simulink model "robot_gripper_vr"  (Simulink 6.5)
settings: Solver=ode45  StartTime=0.0  StopTime=10  RelTol=1e-3
libraries: mblibv1 x39, vrlib x12
settings Model: Creator=arnav  LastModifiedBy=Danek

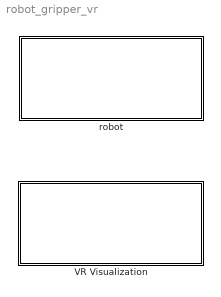
== system robot_gripper_vr ==
  VR Visualization : Subsystem
  robot : Subsystem

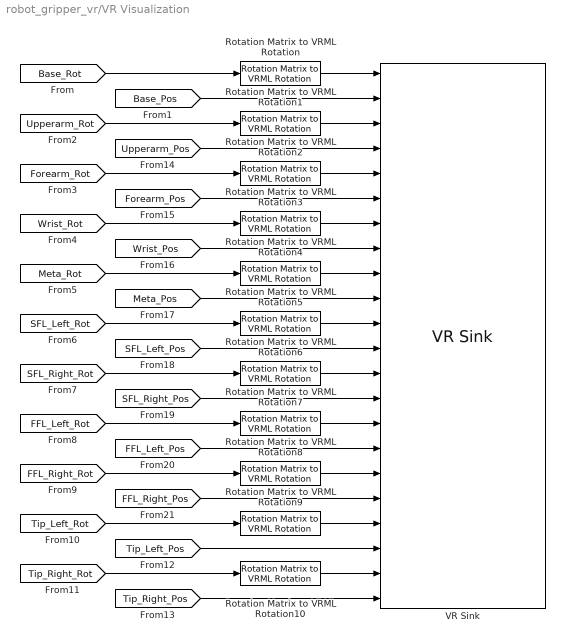
== system robot_gripper_vr/VR Visualization ==
  Rotation Matrix to VRML Rotation{,1..10} (11 alike) : vrlib/Utilities/Rotation Matrix to VRML Rotation  SystemSampleTime=-1  maxzero=1e-12
  VR Sink : vrlib/VR Sink  SampleTime=0.02  ViewEnable=on  RemoteChange=off  RemoteView=on  FieldsWritten=Base.rotation.4.1.double#Base.translation.3.1.double#Upperarm.rotation.4.1.double#Upperarm.translation.3.1.double#Forearm.rotation.4.1.double#Forearm.translation.3.1.double#Wrist.rotation.4.1.double#Wrist.translation.3.1.double#Metacarples.rotation.4.1.double#Metacarples.translation.3.1.double#Fingerlink2_Left.rotation.4.1.double#Fingerlink2_Left.translation.3.1.double#Fingerlink2_Right.rotation.4.1.double#Fingerlink2_Right.translation.3.1.double#Fingerlink1_Left.rotation.4.1.double#Fingerlink1_Left.translation.3.1.double#Fingerlink1_Right.rotation.4.1.double#Fingerlink1_Right.translation.3.1.double#Fingertip_Left.rotation.4.1.double#Fingertip_Left.translation.3.1.double#Fingertip_Right.rotation.4.1.double#Fingertip_Right.translation.3.1.double  WorldFileName=robot_gripper.wrl  WorldDescription=Robot Gripper  AutoView=off  FigureProperties={}
  wires:
  [Base_Rot] -> Rotation Matrix to VRML Rotation/1
  Rotation Matrix to VRML Rotation/1 -> VR Sink/1
  [Base_Pos] -> VR Sink/2
  [Upperarm_Rot] -> Rotation Matrix to VRML Rotation1/1
  [Forearm_Rot] -> Rotation Matrix to VRML Rotation2/1
  [Wrist_Rot] -> Rotation Matrix to VRML Rotation3/1
  [Meta_Rot] -> Rotation Matrix to VRML Rotation4/1
  [SFL_Left_Rot] -> Rotation Matrix to VRML Rotation5/1
  [SFL_Right_Rot] -> Rotation Matrix to VRML Rotation6/1
  [FFL_Left_Rot] -> Rotation Matrix to VRML Rotation7/1
  [FFL_Right_Rot] -> Rotation Matrix to VRML Rotation8/1
  [Tip_Left_Rot] -> Rotation Matrix to VRML Rotation9/1
  [Tip_Right_Rot] -> Rotation Matrix to VRML Rotation10/1
  Rotation Matrix to VRML Rotation1/1 -> VR Sink/3
  Rotation Matrix to VRML Rotation2/1 -> VR Sink/5
  Rotation Matrix to VRML Rotation3/1 -> VR Sink/7
  Rotation Matrix to VRML Rotation4/1 -> VR Sink/9
  Rotation Matrix to VRML Rotation5/1 -> VR Sink/11
  Rotation Matrix to VRML Rotation6/1 -> VR Sink/13
  Rotation Matrix to VRML Rotation7/1 -> VR Sink/15
  Rotation Matrix to VRML Rotation8/1 -> VR Sink/17
  Rotation Matrix to VRML Rotation9/1 -> VR Sink/19
  Rotation Matrix to VRML Rotation10/1 -> VR Sink/21
  [Upperarm_Pos] -> VR Sink/4
  [Forearm_Pos] -> VR Sink/6
  [Wrist_Pos] -> VR Sink/8
  [Meta_Pos] -> VR Sink/10
  [SFL_Left_Pos] -> VR Sink/12
  [SFL_Right_Pos] -> VR Sink/14
  [FFL_Left_Pos] -> VR Sink/16
  [FFL_Right_Pos] -> VR Sink/18
  [Tip_Left_Pos] -> VR Sink/20
  [Tip_Right_Pos] -> VR Sink/22

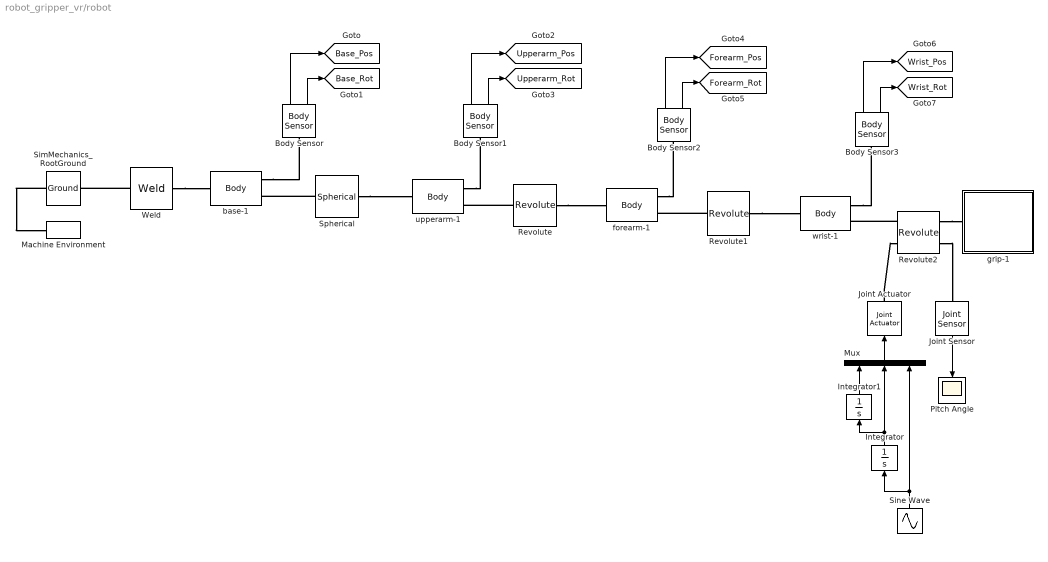
== system robot_gripper_vr/robot ==
  Body Sensor{,1..3} (4 alike) : mblibv1/Sensors &  Actuators/Body Sensor  Orientation=up  DialogController=MECH.DynMechDlgSource  SystemSampleTime=-1  PhysicalDomain=Mechanical  PortType=blob  Muxed=off  Pose=on  Angle=on  AngleUnits=deg  ArcVelocity=off  ArcVelocityUnits=deg/s  ArcAcceleration=off  ArcAccelerationUnits=deg/s^2  CoordPosition=on  CoordPositionUnits=m  Velocity=off  VelocityUnits=m/s  Acceleration=off  AccelerationUnits=m/s^2  Quaternion=on  QuaternionDT=off  QuaternionDDT=off  QuaternionUnits=off  OutputVector=[1]  ActiveIO=on  Width=12  DialogClass=MechanicalSensorBlock  ReferenceFrame=Absolute (World)
  Integrator : Integrator  Orientation=up  InitialCondition=60*pi
  Integrator1 : Integrator  Orientation=up
  Joint Actuator : mblibv1/Sensors &  Actuators/Joint Actuator  Orientation=up  DialogController=MECH.DynMechDlgSource  SystemSampleTime=-1  PhysicalDomain=Mechanical  PortType=blob  ActuationStyle=Motion  AngleUnits=deg  ArcVelocityUnits=deg/s  ArcAccelerationUnits=deg/s^2  CoordPositionUnits=m  VelocityUnits=m/s  AccelerationUnits=m/s^2  ForceUnits=N  TorqueUnits=N*m  ActiveIO=on  Width=3  DialogClass=MechanicalActuatorBlock  Primitive=R1  ReferenceFrame=Absolute (World)
  Joint Sensor : mblibv1/Sensors &  Actuators/Joint Sensor  Orientation=down  DialogController=MECH.DynMechDlgSource  SystemSampleTime=-1  PhysicalDomain=Mechanical  PortType=blob  Muxed=on  Pose=off  Angle=on  AngleUnits=deg  ArcVelocity=off  ArcVelocityUnits=deg/s  ArcAcceleration=off  ArcAccelerationUnits=deg/s^2  CoordPosition=on  CoordPositionUnits=m  Velocity=off  VelocityUnits=m/s  Acceleration=off  AccelerationUnits=m/s^2  Quaternion=on  QuaternionDT=off  QuaternionDDT=off  QuaternionUnits=off  OutputVector=[1]  ActiveIO=on  Width=1  DialogClass=MechanicalSensorBlock  Primitive=R1  Force=off  ForceUnits=N  Torque=off  TorqueUnits=N*m  ReferenceFrame=Absolute (World)  ReactionSensedSide=Base  ReactionReferenceFrame=Absolute (World)  ReactionForce=off  ReactionForceUnits=N  ReactionMoment=off  ReactionMomentUnits=N*m
  Machine Environment : mblibv1/Bodies/Machine Environment  Tag=Factory ground  Orientation=left  DialogController=MECH.DialogSource  SystemSampleTime=-1  PortType=env  PhysicalDomain=Mechanical  DialogTemplateClass=MECH.MachineEnvironment  SyncWhenCopied=off  Gravity=[0 0 0]  GravityUnits=m/s^2  GravityAsSignal=off  Dimensionality=Auto-detect  AnalysisType=Forward dynamics  LinearAssemblyTolerance=1e-2  LinearAssemblyToleranceUnits=m  AngularAssemblyTolerance=1e-1  AngularAssemblyToleranceUnits=rad  ConstraintSolverType=Stabilizing  ConstraintRelTolerance=1e-4  ConstraintAbsTolerance=1e-4  UseRobustSingularityHandling=on  StatePerturbationType=Fixed  PerturbationSize=1e-5  VisualizeMachine=on
  Mux : Mux  Orientation=up  Inputs=3
  Pitch Angle : Scope
      settings: Orientation=down  YMin=-200  YMax=200
  Revolute : mblibv1/Joints/Revolute  DialogController=MECH.DynMechDlgSource  PhysicalDomain=mechanical  SubClassName=Unknown  LeftPortType=blob  RightPortType=blob  LConnTagsString=__newl0  RConnTagsString=__newr0  NumSAPorts=0  CutJoint=off  MarkAsCut=off  Primitives=prismatic  PrimitiveProps=R1$WORLD$[0 1 0]$revolute  DialogClass=JointBlock  R1Axis=[0 1 0]
  Revolute1 : mblibv1/Joints/Revolute  DialogController=MECH.DynMechDlgSource  PhysicalDomain=mechanical  SubClassName=Unknown  LeftPortType=blob  RightPortType=blob  LConnTagsString=__newl0  RConnTagsString=__newr0  NumSAPorts=0  CutJoint=off  MarkAsCut=off  Primitives=prismatic  PrimitiveProps=R1$World$[0 0 1]$revolute  DialogClass=JointBlock  R1Axis=[0 0 1]
  Revolute2 : mblibv1/Joints/Revolute  DialogController=MECH.DynMechDlgSource  PhysicalDomain=mechanical  SubClassName=Unknown  LeftPortType=blob  RightPortType=blob  LConnTagsString=__newl0|SA1  RConnTagsString=__newr0|SA1  NumSAPorts=2  CutJoint=off  MarkAsCut=off  Primitives=prismatic  PrimitiveProps=R1$World$[1 0 0]$revolute  DialogClass=JointBlock  R1Axis=[1 0 0]
  SimMechanics_RootGround : mblibv1/Bodies/Ground  DialogController=MECH.DynMechDlgSource  SystemSampleTime=-1  LeftPortType=env  RightPortType=workingframe  PhysicalDomain=Mechanical  DialogClass=GroundBlock  CoordPosition=[0 0 0]  CoordPositionUnits=m  StateVectorMgrId=-1  MachineId=[2 0]  ShowEnvPort=on
  Sine Wave : Sin  Orientation=up  Amplitude=60*pi*pi  Frequency=60  SampleTime=0
  Spherical : mblibv1/Joints/Spherical  DialogController=MECH.DynMechDlgSource  PhysicalDomain=mechanical  SubClassName=Unknown  LeftPortType=blob  RightPortType=blob  LConnTagsString=__newl0  RConnTagsString=__newr0  NumSAPorts=0  CutJoint=off  MarkAsCut=off  Primitives=spherical  PrimitiveProps=S$WORLD$[0 0 0]$spherical  DialogClass=JointBlock  SAxis=[0 0 0]
  Weld : mblibv1/Joints/Weld  DialogController=MECH.DynMechDlgSource  PhysicalDomain=mechanical  SubClassName=Unknown  LeftPortType=blob  RightPortType=blob  LConnTagsString=__newl0  RConnTagsString=__newr0  NumSAPorts=0  CutJoint=off  MarkAsCut=off  Primitives=weld  PrimitiveProps=W$WORLD$[0 0 0]$weld  DialogClass=JointBlock  WAxis=[0 0 0]
  base-1 : mblibv1/Bodies/Body  DialogController=MECH.DynMechDlgSource  PhysicalDomain=mechanical  SubClassName=Unknown  LeftPortType=workingframe  RightPortType=workingframe  LConnTagsString=CS3  RConnTagsString=CS1|CS2  DialogClass=MechanicalBodyBlock  Mass=9.4647  MassUnits=kg  InertiaUnits=kg*m^2  Inertia=[0.019805 0.00027282 5.3173e-009;0.00027282 0.040113 4.235e-009;5.3173e-009 4.235e-009 0.027428]  Shape=robot - base-1  ShapeDims=[1 1]  ShapeUnits=m  ShapeUse=false  Density=1  DensityUnits=kg/m^3  DensityUse=false  CG=Right$CG$[-0.028401 0.023565 1.9023e-008]$WORLD$WORLD$m$[1 0 0;0 1 0;0 0 1]$3x3 Transform$rad$WORLD$false  WorkingFrames=Right$CS1$[0 0 0]$WORLD$WORLD$m$[1 0 0;0 1 0;0 0 1]$3x3 Transform$rad$WORLD$true#Right$CS2$[-0.0127 0.1322 0]$WORLD$WORLD$m$[1 0 0;0 1 0;0 0 1]$3x3 Transform$rad$WORLD$true#Left$CS3$[0 0 0]$WORLD$WORLD$m$[1 0 0;0 1 0;0 0 1]$3x3 Transform$rad$WORLD$true  CGPos=[-0.028401 0.023565 1.9023e-008]  CGRot=[1 0 0;0 1 0;0 0 1]  CS0Pos=[]  CS0Rot=[]  CS1Pos=[0 0 0]  CS1Rot=[1 0 0;0 1 0;0 0 1]  CS2Pos=[-0.0127 0.1322 0]  CS2Rot=[1 0 0;0 1 0;0 0 1]  CS3Pos=[0 0 0]  CS3Rot=[1 0 0;0 1 0;0 0 1]  CS4Pos=[]  CS4Rot=[]  CS5Pos=[]  CS5Rot=[]  CS6Pos=[]  CS6Rot=[]  CS7Pos=[]  CS7Rot=[]  CS8Pos=[]  CS8Rot=[]  CS9Pos=[]  CS9Rot=[]  CS10Pos=[]  CS10Rot=[]  CS11Pos=[]  CS11Rot=[]  CS12Pos=[]  CS12Rot=[]  CS13Pos=[]  CS13Rot=[]  CS14Pos=[]  CS14Rot=[]  CS15Pos=[]  CS15Rot=[]  CS16Pos=[]  CS16Rot=[]  CS17Pos=[]  CS17Rot=[]  CS18Pos=[]  CS18Rot=[]  CS19Pos=[]  CS19Rot=[]  CS20Pos=[]  CS20Rot=[]
  forearm-1 : mblibv1/Bodies/Body  DialogController=MECH.DynMechDlgSource  PhysicalDomain=mechanical  SubClassName=Unknown  LeftPortType=workingframe  RightPortType=workingframe  LConnTagsString=CS2  RConnTagsString=CS4|CS3  DialogClass=MechanicalBodyBlock  Mass=1.0045  MassUnits=kg  InertiaUnits=kg*m^2  Inertia=[0.00025695 -1.1574e-007 8.8892e-012;-1.1574e-007 0.0011733 6.7457e-012;8.8892e-012 6.7457e-012 0.0010899]  Shape=robot - forearm-1  ShapeDims=[1 1]  ShapeUnits=m  ShapeUse=false  Density=1  DensityUnits=kg/m^3  DensityUse=false  CG=Right$CG$[0.14456 0.13136 -2.1677e-010]$WORLD$WORLD$m$[1 0 0;0 1 0;0 0 1]$3x3 Transform$rad$WORLD$false  WorkingFrames=Right$CS4$[0 0 0]$WORLD$WORLD$m$[1 0 0;0 1 0;0 0 1]$3x3 Transform$rad$WORLD$true#Left$CS2$[0.08763 0.13118 0]$WORLD$WORLD$m$[1 0 0;0 1 0;0 0 1]$3x3 Transform$rad$WORLD$true#Right$CS3$[0.19685 0.13118 0]$WORLD$WORLD$m$[1 0 0;0 1 0;0 0 1]$3x3 Transform$rad$WORLD$true#Right$CS1$[0.10414 0.13118 0]$WORLD$WORLD$m$[1 0 0;0 1 0;0 0 1]$3x3 Transform$rad$WORLD$false  CGPos=[0.14456 0.13136 -2.1677e-010]  CGRot=[1 0 0;0 1 0;0 0 1]  CS0Pos=[]  CS0Rot=[]  CS1Pos=[0.10414 0.13118 0]  CS1Rot=[1 0 0;0 1 0;0 0 1]  CS2Pos=[0.08763 0.13118 0]  CS2Rot=[1 0 0;0 1 0;0 0 1]  CS3Pos=[0.19685 0.13118 0]  CS3Rot=[1 0 0;0 1 0;0 0 1]  CS4Pos=[0 0 0]  CS4Rot=[1 0 0;0 1 0;0 0 1]  CS5Pos=[]  CS5Rot=[]  CS6Pos=[]  CS6Rot=[]  CS7Pos=[]  CS7Rot=[]  CS8Pos=[]  CS8Rot=[]  CS9Pos=[]  CS9Rot=[]  CS10Pos=[]  CS10Rot=[]  CS11Pos=[]  CS11Rot=[]  CS12Pos=[]  CS12Rot=[]  CS13Pos=[]  CS13Rot=[]  CS14Pos=[]  CS14Rot=[]  CS15Pos=[]  CS15Rot=[]  CS16Pos=[]  CS16Rot=[]  CS17Pos=[]  CS17Rot=[]  CS18Pos=[]  CS18Rot=[]  CS19Pos=[]  CS19Rot=[]  CS20Pos=[]  CS20Rot=[]
  grip-1 : Subsystem
  upperarm-1 : mblibv1/Bodies/Body  DialogController=MECH.DynMechDlgSource  PhysicalDomain=mechanical  SubClassName=Unknown  LeftPortType=workingframe  RightPortType=workingframe  LConnTagsString=CS3  RConnTagsString=CS4|CS2  DialogClass=MechanicalBodyBlock  Mass=0.80158  MassUnits=kg  InertiaUnits=kg*m^2  Inertia=[0.00065457 -6.3977e-005 5.5009e-009;-6.3977e-005 0.0024771 2.4583e-009;5.5009e-009 2.4583e-009 0.0023575]  Shape=robot - upperarm-1  ShapeDims=[1 1]  ShapeUnits=m  ShapeUse=false  Density=1  DensityUnits=kg/m^3  DensityUse=false  CG=Right$CG$[0.013784 0.13487 -1.5235e-007]$WORLD$WORLD$m$[1 0 0;0 1 0;0 0 1]$3x3 Transform$rad$WORLD$false  WorkingFrames=Right$CS4$[0 0 0]$WORLD$WORLD$m$[1 0 0;0 1 0;0 0 1]$3x3 Transform$rad$WORLD$true#Right$CS2$[0.08763 0.13118 0]$WORLD$WORLD$m$[1 0 0;0 1 0;0 0 1]$3x3 Transform$rad$WORLD$true#Left$CS3$[-0.0127 0.1322 0]$WORLD$WORLD$m$[1 0 0;0 1 0;0 0 1]$3x3 Transform$rad$WORLD$true#Right$CS1$[-0.0127 0.1322 0]$WORLD$WORLD$m$[1 0 0;0 1 0;0 0 1]$3x3 Transform$rad$WORLD$false  CGPos=[0.013784 0.13487 -1.5235e-007]  CGRot=[1 0 0;0 1 0;0 0 1]  CS0Pos=[]  CS0Rot=[]  CS1Pos=[-0.0127 0.1322 0]  CS1Rot=[1 0 0;0 1 0;0 0 1]  CS2Pos=[0.08763 0.13118 0]  CS2Rot=[1 0 0;0 1 0;0 0 1]  CS3Pos=[-0.0127 0.1322 0]  CS3Rot=[1 0 0;0 1 0;0 0 1]  CS4Pos=[0 0 0]  CS4Rot=[1 0 0;0 1 0;0 0 1]  CS5Pos=[]  CS5Rot=[]  CS6Pos=[]  CS6Rot=[]  CS7Pos=[]  CS7Rot=[]  CS8Pos=[]  CS8Rot=[]  CS9Pos=[]  CS9Rot=[]  CS10Pos=[]  CS10Rot=[]  CS11Pos=[]  CS11Rot=[]  CS12Pos=[]  CS12Rot=[]  CS13Pos=[]  CS13Rot=[]  CS14Pos=[]  CS14Rot=[]  CS15Pos=[]  CS15Rot=[]  CS16Pos=[]  CS16Rot=[]  CS17Pos=[]  CS17Rot=[]  CS18Pos=[]  CS18Rot=[]  CS19Pos=[]  CS19Rot=[]  CS20Pos=[]  CS20Rot=[]
  wrist-1 : mblibv1/Bodies/Body  DialogController=MECH.DynMechDlgSource  PhysicalDomain=mechanical  SubClassName=Unknown  LeftPortType=workingframe  RightPortType=workingframe  LConnTagsString=CS2  RConnTagsString=CS4|CS3  DialogClass=MechanicalBodyBlock  Mass=0.15168  MassUnits=kg  InertiaUnits=kg*m^2  Inertia=[2.7107e-005 -4.382e-012 -5.6539e-012;-4.382e-012 4.6303e-005 1.5497e-011;-5.6539e-012 1.5497e-011 3.8794e-005]  Shape=robot - wrist-1  ShapeDims=[1 1]  ShapeUnits=m  ShapeUse=false  Density=1  DensityUnits=kg/m^3  DensityUse=false  CG=Right$CG$[0.20752 0.13118 2.0847e-009]$WORLD$WORLD$m$[1 0 0;0 1 0;0 0 1]$3x3 Transform$rad$WORLD$false  WorkingFrames=Right$CS4$[0 0 0]$WORLD$WORLD$m$[1 0 0;0 1 0;0 0 1]$3x3 Transform$rad$WORLD$true#Left$CS2$[0.19685 0.13118 0]$WORLD$WORLD$m$[1 0 0;0 1 0;0 0 1]$3x3 Transform$rad$WORLD$true#Right$CS3$[0.22733 0.13118 0]$WORLD$WORLD$m$[1 0 0;0 1 0;0 0 1]$3x3 Transform$rad$WORLD$true#Right$CS1$[0.21209 0.13118 0]$WORLD$WORLD$m$[1 0 0;0 1 0;0 0 1]$3x3 Transform$rad$WORLD$false  CGPos=[0.20752 0.13118 2.0847e-009]  CGRot=[1 0 0;0 1 0;0 0 1]  CS0Pos=[]  CS0Rot=[]  CS1Pos=[0.21209 0.13118 0]  CS1Rot=[1 0 0;0 1 0;0 0 1]  CS2Pos=[0.19685 0.13118 0]  CS2Rot=[1 0 0;0 1 0;0 0 1]  CS3Pos=[0.22733 0.13118 0]  CS3Rot=[1 0 0;0 1 0;0 0 1]  CS4Pos=[0 0 0]  CS4Rot=[1 0 0;0 1 0;0 0 1]  CS5Pos=[]  CS5Rot=[]  CS6Pos=[]  CS6Rot=[]  CS7Pos=[]  CS7Rot=[]  CS8Pos=[]  CS8Rot=[]  CS9Pos=[]  CS9Rot=[]  CS10Pos=[]  CS10Rot=[]  CS11Pos=[]  CS11Rot=[]  CS12Pos=[]  CS12Rot=[]  CS13Pos=[]  CS13Rot=[]  CS14Pos=[]  CS14Rot=[]  CS15Pos=[]  CS15Rot=[]  CS16Pos=[]  CS16Rot=[]  CS17Pos=[]  CS17Rot=[]  CS18Pos=[]  CS18Rot=[]  CS19Pos=[]  CS19Rot=[]  CS20Pos=[]  CS20Rot=[]
  tag scope: Base_Pos=global, Base_Rot=global, Forearm_Pos=global, Forearm_Rot=global, Upperarm_Pos=global, Upperarm_Rot=global, Wrist_Pos=global, Wrist_Rot=global
  wires:
  Mux/1 -> Joint Actuator/1
  Body Sensor/1 -> [Base_Pos]
  Body Sensor/2 -> [Base_Rot]
  Body Sensor1/1 -> [Upperarm_Pos]
  Body Sensor1/2 -> [Upperarm_Rot]
  Body Sensor2/1 -> [Forearm_Pos]
  Body Sensor2/2 -> [Forearm_Rot]
  Body Sensor3/1 -> [Wrist_Pos]
  Body Sensor3/2 -> [Wrist_Rot]
  Integrator/1 -> Integrator1/1, Mux/2
  Integrator1/1 -> Mux/1
  Joint Sensor/1 -> Pitch Angle/1
  Sine Wave/1 -> Mux/3, Integrator/1
  connections:
  Weld/LConn1 -- SimMechanics_RootGround/RConn1
  Weld/RConn1 -- base-1/LConn1
  Revolute/LConn1 -- upperarm-1/RConn2
  Revolute/RConn1 -- forearm-1/LConn1
  Revolute1/LConn1 -- forearm-1/RConn2
  Revolute1/RConn1 -- wrist-1/LConn1
  Revolute2/LConn1 -- wrist-1/RConn2
  Revolute2/RConn1 -- grip-1/LConn1
  Spherical/LConn1 -- base-1/RConn2
  Spherical/RConn1 -- upperarm-1/LConn1
  SimMechanics_RootGround/LConn1 -- Machine Environment/RConn1
  upperarm-1/RConn1 -- Body Sensor1/LConn1
  forearm-1/RConn1 -- Body Sensor2/LConn1
  wrist-1/RConn1 -- Body Sensor3/LConn1
  base-1/RConn1 -- Body Sensor/LConn1
  Joint Actuator/RConn1 -- Revolute2/LConn2
  Revolute2/RConn2 -- Joint Sensor/LConn1

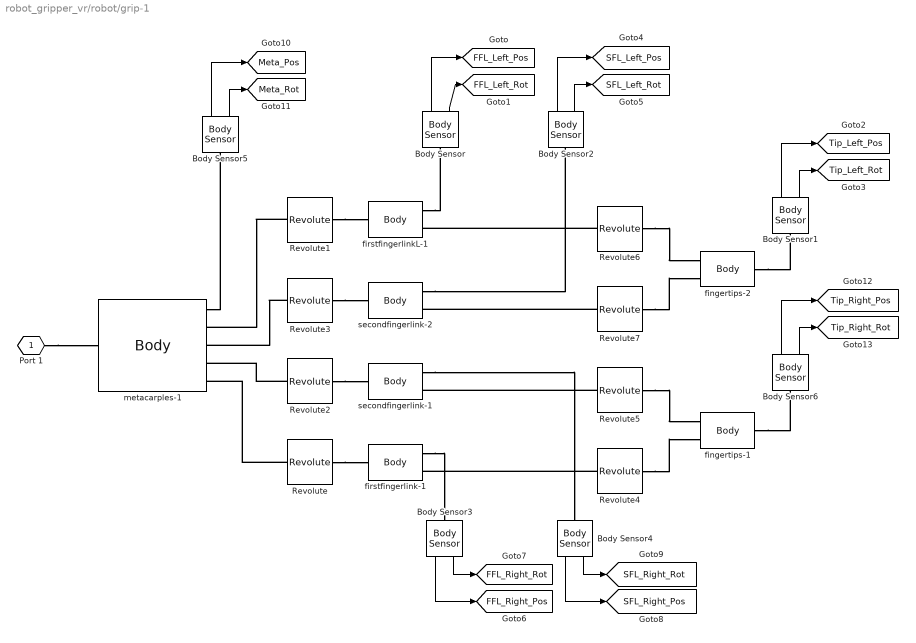
== system robot_gripper_vr/robot/grip-1 ==
  Body Sensor{,1..2,5..6} (5 alike) : mblibv1/Sensors &  Actuators/Body Sensor  Orientation=up  DialogController=MECH.DynMechDlgSource  SystemSampleTime=-1  PhysicalDomain=Mechanical  PortType=blob  Muxed=off  Pose=on  Angle=on  AngleUnits=deg  ArcVelocity=off  ArcVelocityUnits=deg/s  ArcAcceleration=off  ArcAccelerationUnits=deg/s^2  CoordPosition=on  CoordPositionUnits=m  Velocity=off  VelocityUnits=m/s  Acceleration=off  AccelerationUnits=m/s^2  Quaternion=on  QuaternionDT=off  QuaternionDDT=off  QuaternionUnits=off  OutputVector=[1]  ActiveIO=on  Width=12  DialogClass=MechanicalSensorBlock  ReferenceFrame=Absolute (World)
  Body Sensor3 : mblibv1/Sensors &  Actuators/Body Sensor  Orientation=down  DialogController=MECH.DynMechDlgSource  SystemSampleTime=-1  PhysicalDomain=Mechanical  PortType=blob  Muxed=off  Pose=on  Angle=on  AngleUnits=deg  ArcVelocity=off  ArcVelocityUnits=deg/s  ArcAcceleration=off  ArcAccelerationUnits=deg/s^2  CoordPosition=on  CoordPositionUnits=m  Velocity=off  VelocityUnits=m/s  Acceleration=off  AccelerationUnits=m/s^2  Quaternion=on  QuaternionDT=off  QuaternionDDT=off  QuaternionUnits=off  OutputVector=[1]  ActiveIO=on  Width=12  DialogClass=MechanicalSensorBlock  ReferenceFrame=Absolute (World)
  Body Sensor4 : mblibv1/Sensors &  Actuators/Body Sensor  Orientation=down  DialogController=MECH.DynMechDlgSource  SystemSampleTime=-1  PhysicalDomain=Mechanical  PortType=blob  Muxed=off  Pose=on  Angle=on  AngleUnits=deg  ArcVelocity=off  ArcVelocityUnits=deg/s  ArcAcceleration=off  ArcAccelerationUnits=deg/s^2  CoordPosition=on  CoordPositionUnits=m  Velocity=off  VelocityUnits=m/s  Acceleration=off  AccelerationUnits=m/s^2  Quaternion=on  QuaternionDT=off  QuaternionDDT=off  QuaternionUnits=off  OutputVector=[1]  ActiveIO=on  Width=12  DialogClass=MechanicalSensorBlock  ReferenceFrame=Absolute (World)
  Revolute{,1..5} (6 alike) : mblibv1/Joints/Revolute  DialogController=MECH.DynMechDlgSource  PhysicalDomain=mechanical  SubClassName=Unknown  LeftPortType=blob  RightPortType=blob  LConnTagsString=__newl0  RConnTagsString=__newr0  NumSAPorts=0  CutJoint=off  MarkAsCut=off  Primitives=prismatic  PrimitiveProps=R1$WORLD$[0 1 0]$revolute  DialogClass=JointBlock  R1Axis=[0 1 0]
  Revolute6 : mblibv1/Joints/Revolute  DialogController=MECH.DynMechDlgSource  PhysicalDomain=mechanical  SubClassName=Unknown  LeftPortType=blob  RightPortType=blob  LConnTagsString=__newl0  RConnTagsString=__newr0  NumSAPorts=0  CutJoint=off  MarkAsCut=off  Primitives=prismatic  PrimitiveProps=R1$WORLD$[0 -1 0]$revolute  DialogClass=JointBlock  R1Axis=[0 -1 0]
  Revolute7 : mblibv1/Joints/Revolute  DialogController=MECH.DynMechDlgSource  PhysicalDomain=mechanical  SubClassName=Unknown  LeftPortType=blob  RightPortType=blob  LConnTagsString=__newl0  RConnTagsString=__newr0  NumSAPorts=0  CutJoint=off  MarkAsCut=off  Primitives=prismatic  PrimitiveProps=R1$WORLD$[0 -1 0]$revolute  DialogClass=JointBlock  R1Axis=[0 -1 0]
  fingertips-1 : mblibv1/Bodies/Body  DialogController=MECH.DynMechDlgSource  PhysicalDomain=mechanical  SubClassName=Unknown  LeftPortType=workingframe  RightPortType=workingframe  LConnTagsString=CS3|CS2  RConnTagsString=CS4  DialogClass=MechanicalBodyBlock  Mass=0.025178  MassUnits=kg  InertiaUnits=kg*m^2  Inertia=[6.5444e-007 3.3719e-010 -1.0605e-006;3.3719e-010 4.9015e-006 -1.4396e-010;-1.0605e-006 -1.4396e-010 4.6494e-006]  Shape=robot - grip-1 fingertips-1  ShapeDims=[1 1]  ShapeUnits=m  ShapeUse=false  Density=1  DensityUnits=kg/m^3  DensityUse=false  CG=Right$CG$[0.30147 0.13118 0.028955]$WORLD$WORLD$m$[0.94 0 -0.34117;0 1 0;0.34117 0 0.94]$3x3 Transform$rad$WORLD$false  WorkingFrames=Right$CS4$[0 0 0]$WORLD$WORLD$m$[1 0 0;0 1 0;0 0 1]$3x3 Transform$rad$WORLD$true#Left$CS3$[0.29493 0.13118 0.023689]$WORLD$WORLD$m$[1 0 0;0 1 0;0 0 1]$3x3 Transform$rad$WORLD$true#Left$CS2$[0.27228 0.13118 0.026422]$WORLD$WORLD$m$[1 0 0;0 1 0;0 0 1]$3x3 Transform$rad$WORLD$true#Right$CS1$[0.29902 0.13118 0.027332]$WORLD$WORLD$m$[1 0 0;0 1 0;0 0 1]$3x3 Transform$rad$WORLD$false  CGPos=[0.30147 0.13118 0.028955]  CGRot=[0.94 0 -0.34117;0 1 0;0.34117 0 0.94]  CS0Pos=[]  CS0Rot=[]  CS1Pos=[0.29902 0.13118 0.027332]  CS1Rot=[1 0 0;0 1 0;0 0 1]  CS2Pos=[0.27228 0.13118 0.026422]  CS2Rot=[1 0 0;0 1 0;0 0 1]  CS3Pos=[0.29493 0.13118 0.023689]  CS3Rot=[1 0 0;0 1 0;0 0 1]  CS4Pos=[0 0 0]  CS4Rot=[1 0 0;0 1 0;0 0 1]  CS5Pos=[]  CS5Rot=[]  CS6Pos=[]  CS6Rot=[]  CS7Pos=[]  CS7Rot=[]  CS8Pos=[]  CS8Rot=[]  CS9Pos=[]  CS9Rot=[]  CS10Pos=[]  CS10Rot=[]  CS11Pos=[]  CS11Rot=[]  CS12Pos=[]  CS12Rot=[]  CS13Pos=[]  CS13Rot=[]  CS14Pos=[]  CS14Rot=[]  CS15Pos=[]  CS15Rot=[]  CS16Pos=[]  CS16Rot=[]  CS17Pos=[]  CS17Rot=[]  CS18Pos=[]  CS18Rot=[]  CS19Pos=[]  CS19Rot=[]  CS20Pos=[]  CS20Rot=[]
  fingertips-2 : mblibv1/Bodies/Body  DialogController=MECH.DynMechDlgSource  PhysicalDomain=mechanical  SubClassName=Unknown  LeftPortType=workingframe  RightPortType=workingframe  LConnTagsString=CS2|CS3  RConnTagsString=CS4  DialogClass=MechanicalBodyBlock  Mass=0.025178  MassUnits=kg  InertiaUnits=kg*m^2  Inertia=[6.5444e-007 3.3719e-010 -1.0605e-006;3.3719e-010 4.9015e-006 -1.4396e-010;-1.0605e-006 -1.4396e-010 4.6494e-006]  Shape=robot - grip-1 fingertips-2  ShapeDims=[1 1]  ShapeUnits=m  ShapeUse=false  Density=1  DensityUnits=kg/m^3  DensityUse=false  CG=Right$CG$[0.30147 0.13118 -0.028955]$WORLD$WORLD$m$[0.94 0 -0.34117;0 -1 0;-0.34117 0 -0.94]$3x3 Transform$rad$WORLD$false  WorkingFrames=Right$CS4$[0 0 0]$WORLD$WORLD$m$[1 0 0;0 1 0;0 0 1]$3x3 Transform$rad$WORLD$true#Left$CS2$[0.27228 0.13118 -0.026422]$WORLD$WORLD$m$[1 0 0;0 1 0;0 0 1]$3x3 Transform$rad$WORLD$true#Left$CS3$[0.29493 0.13118 -0.023689]$WORLD$WORLD$m$[1 0 0;0 1 0;0 0 1]$3x3 Transform$rad$WORLD$true#Right$CS1$[0.29902 0.13118 -0.027332]$WORLD$WORLD$m$[1 0 0;0 1 0;0 0 1]$3x3 Transform$rad$WORLD$false  CGPos=[0.30147 0.13118 -0.028955]  CGRot=[0.94 0 -0.34117;0 -1 0;-0.34117 0 -0.94]  CS0Pos=[]  CS0Rot=[]  CS1Pos=[0.29902 0.13118 -0.027332]  CS1Rot=[1 0 0;0 1 0;0 0 1]  CS2Pos=[0.27228 0.13118 -0.026422]  CS2Rot=[1 0 0;0 1 0;0 0 1]  CS3Pos=[0.29493 0.13118 -0.023689]  CS3Rot=[1 0 0;0 1 0;0 0 1]  CS4Pos=[0 0 0]  CS4Rot=[1 0 0;0 1 0;0 0 1]  CS5Pos=[]  CS5Rot=[]  CS6Pos=[]  CS6Rot=[]  CS7Pos=[]  CS7Rot=[]  CS8Pos=[]  CS8Rot=[]  CS9Pos=[]  CS9Rot=[]  CS10Pos=[]  CS10Rot=[]  CS11Pos=[]  CS11Rot=[]  CS12Pos=[]  CS12Rot=[]  CS13Pos=[]  CS13Rot=[]  CS14Pos=[]  CS14Rot=[]  CS15Pos=[]  CS15Rot=[]  CS16Pos=[]  CS16Rot=[]  CS17Pos=[]  CS17Rot=[]  CS18Pos=[]  CS18Rot=[]  CS19Pos=[]  CS19Rot=[]  CS20Pos=[]  CS20Rot=[]
  firstfingerlink-1 : mblibv1/Bodies/Body  DialogController=MECH.DynMechDlgSource  PhysicalDomain=mechanical  SubClassName=Unknown  LeftPortType=workingframe  RightPortType=workingframe  LConnTagsString=CS2  RConnTagsString=CS4|CS3  DialogClass=MechanicalBodyBlock  Mass=0.0072753  MassUnits=kg  InertiaUnits=kg*m^2  Inertia=[1.3879e-007 2.8825e-008 3.0548e-008;2.8825e-008 5.4293e-007 9.6984e-009;3.0548e-008 9.6984e-009 5.7607e-007]  Shape=robot - grip-1 firstfingerlink-1  ShapeDims=[1 1]  ShapeUnits=m  ShapeUse=false  Density=1  DensityUnits=kg/m^3  DensityUse=false  CG=Right$CG$[0.2636 0.13052 0.018155]$WORLD$WORLD$m$[0.70711 0 -0.70711;0 1 0;0.70711 0 0.70711]$3x3 Transform$rad$WORLD$false  WorkingFrames=Right$CS4$[0 0 0]$WORLD$WORLD$m$[1 0 0;0 1 0;0 0 1]$3x3 Transform$rad$WORLD$true#Left$CS2$[0.2624 0.13118 0.011156]$WORLD$WORLD$m$[1 0 0;0 1 0;0 0 1]$3x3 Transform$rad$WORLD$true#Right$CS3$[0.27228 0.13118 0.026422]$WORLD$WORLD$m$[1 0 0;0 1 0;0 0 1]$3x3 Transform$rad$WORLD$true#Right$CS1$[0.2624 0.13118 0.011156]$WORLD$WORLD$m$[1 0 0;0 1 0;0 0 1]$3x3 Transform$rad$WORLD$false  CGPos=[0.2636 0.13052 0.018155]  CGRot=[0.70711 0 -0.70711;0 1 0;0.70711 0 0.70711]  CS0Pos=[]  CS0Rot=[]  CS1Pos=[0.2624 0.13118 0.011156]  CS1Rot=[1 0 0;0 1 0;0 0 1]  CS2Pos=[0.2624 0.13118 0.011156]  CS2Rot=[1 0 0;0 1 0;0 0 1]  CS3Pos=[0.27228 0.13118 0.026422]  CS3Rot=[1 0 0;0 1 0;0 0 1]  CS4Pos=[0 0 0]  CS4Rot=[1 0 0;0 1 0;0 0 1]  CS5Pos=[]  CS5Rot=[]  CS6Pos=[]  CS6Rot=[]  CS7Pos=[]  CS7Rot=[]  CS8Pos=[]  CS8Rot=[]  CS9Pos=[]  CS9Rot=[]  CS10Pos=[]  CS10Rot=[]  CS11Pos=[]  CS11Rot=[]  CS12Pos=[]  CS12Rot=[]  CS13Pos=[]  CS13Rot=[]  CS14Pos=[]  CS14Rot=[]  CS15Pos=[]  CS15Rot=[]  CS16Pos=[]  CS16Rot=[]  CS17Pos=[]  CS17Rot=[]  CS18Pos=[]  CS18Rot=[]  CS19Pos=[]  CS19Rot=[]  CS20Pos=[]  CS20Rot=[]
  firstfingerlinkL-1 : mblibv1/Bodies/Body  DialogController=MECH.DynMechDlgSource  PhysicalDomain=mechanical  SubClassName=Unknown  LeftPortType=workingframe  RightPortType=workingframe  LConnTagsString=CS2  RConnTagsString=CS4|CS3  DialogClass=MechanicalBodyBlock  Mass=0.0072753  MassUnits=kg  InertiaUnits=kg*m^2  Inertia=[1.3879e-007 2.8825e-008 -3.0547e-008;2.8825e-008 5.4293e-007 -9.6984e-009;-3.0547e-008 -9.6984e-009 5.7607e-007]  Shape=robot - grip-1 firstfingerlinkL-1  ShapeDims=[1 1]  ShapeUnits=m  ShapeUse=false  Density=1  DensityUnits=kg/m^3  DensityUse=false  CG=Right$CG$[0.2636 0.13052 -0.018155]$WORLD$WORLD$m$[0.70711 0 0.70711;0 1 0;-0.70711 0 0.70711]$3x3 Transform$rad$WORLD$false  WorkingFrames=Right$CS4$[0 0 0]$WORLD$WORLD$m$[1 0 0;0 1 0;0 0 1]$3x3 Transform$rad$WORLD$true#Left$CS2$[0.2624 0.13118 -0.011156]$WORLD$WORLD$m$[1 0 0;0 1 0;0 0 1]$3x3 Transform$rad$WORLD$true#Right$CS3$[0.27228 0.13118 -0.026422]$WORLD$WORLD$m$[1 0 0;0 1 0;0 0 1]$3x3 Transform$rad$WORLD$true#Right$CS1$[0.2624 0.13118 -0.011156]$WORLD$WORLD$m$[1 0 0;0 1 0;0 0 1]$3x3 Transform$rad$WORLD$false  CGPos=[0.2636 0.13052 -0.018155]  CGRot=[0.70711 0 0.70711;0 1 0;-0.70711 0 0.70711]  CS0Pos=[]  CS0Rot=[]  CS1Pos=[0.2624 0.13118 -0.011156]  CS1Rot=[1 0 0;0 1 0;0 0 1]  CS2Pos=[0.2624 0.13118 -0.011156]  CS2Rot=[1 0 0;0 1 0;0 0 1]  CS3Pos=[0.27228 0.13118 -0.026422]  CS3Rot=[1 0 0;0 1 0;0 0 1]  CS4Pos=[0 0 0]  CS4Rot=[1 0 0;0 1 0;0 0 1]  CS5Pos=[]  CS5Rot=[]  CS6Pos=[]  CS6Rot=[]  CS7Pos=[]  CS7Rot=[]  CS8Pos=[]  CS8Rot=[]  CS9Pos=[]  CS9Rot=[]  CS10Pos=[]  CS10Rot=[]  CS11Pos=[]  CS11Rot=[]  CS12Pos=[]  CS12Rot=[]  CS13Pos=[]  CS13Rot=[]  CS14Pos=[]  CS14Rot=[]  CS15Pos=[]  CS15Rot=[]  CS16Pos=[]  CS16Rot=[]  CS17Pos=[]  CS17Rot=[]  CS18Pos=[]  CS18Rot=[]  CS19Pos=[]  CS19Rot=[]  CS20Pos=[]  CS20Rot=[]
  metacarples-1 : mblibv1/Bodies/Body  DialogController=MECH.DynMechDlgSource  PhysicalDomain=mechanical  SubClassName=Unknown  LeftPortType=workingframe  RightPortType=workingframe  LConnTagsString=CS2  RConnTagsString=CS7|CS4|CS6|CS5|CS3  DialogClass=MechanicalBodyBlock  Mass=0.29497  MassUnits=kg  InertiaUnits=kg*m^2  Inertia=[7.8711e-005 -1.8885e-011 -2.8356e-012;-1.8885e-011 8.5557e-005 9.0013e-012;-2.8356e-012 9.0013e-012 7.0503e-005]  Shape=robot - grip-1 metacarples-1  ShapeDims=[1 1]  ShapeUnits=m  ShapeUse=false  Density=1  DensityUnits=kg/m^3  DensityUse=false  CG=Right$CG$[0.25156 0.13118 7.829e-009]$WORLD$WORLD$m$[1 0 0;0 1 0;0 0 1]$3x3 Transform$rad$WORLD$false  WorkingFrames=Right$CS7$[0 0 0]$WORLD$WORLD$m$[1 0 0;0 1 0;0 0 1]$3x3 Transform$rad$WORLD$true#Right$CS4$[0.2624 0.13118 -0.011156]$WORLD$WORLD$m$[1 0 0;0 1 0;0 0 1]$3x3 Transform$rad$WORLD$true#Right$CS6$[0.28286 0.13118 -0.0054884]$WORLD$WORLD$m$[1 0 0;0 1 0;0 0 1]$3x3 Transform$rad$WORLD$true#Left$CS2$[0.22733 0.13118 0]$WORLD$WORLD$m$[1 0 0;0 1 0;0 0 1]$3x3 Transform$rad$WORLD$true#Right$CS5$[0.28286 0.13118 0.0054884]$WORLD$WORLD$m$[1 0 0;0 1 0;0 0 1]$3x3 Transform$rad$WORLD$true#Right$CS3$[0.2624 0.13118 0.011156]$WORLD$WORLD$m$[1 0 0;0 1 0;0 0 1]$3x3 Transform$rad$WORLD$true#Right$CS1$[0.24638 0.13118 0]$WORLD$WORLD$m$[1 0 0;0 1 0;0 0 1]$3x3 Transform$rad$WORLD$false  CGPos=[0.25156 0.13118 7.829e-009]  CGRot=[1 0 0;0 1 0;0 0 1]  CS0Pos=[]  CS0Rot=[]  CS1Pos=[0.24638 0.13118 0]  CS1Rot=[1 0 0;0 1 0;0 0 1]  CS2Pos=[0.22733 0.13118 0]  CS2Rot=[1 0 0;0 1 0;0 0 1]  CS3Pos=[0.2624 0.13118 0.011156]  CS3Rot=[1 0 0;0 1 0;0 0 1]  CS4Pos=[0.2624 0.13118 -0.011156]  CS4Rot=[1 0 0;0 1 0;0 0 1]  CS5Pos=[0.28286 0.13118 0.0054884]  CS5Rot=[1 0 0;0 1 0;0 0 1]  CS6Pos=[0.28286 0.13118 -0.0054884]  CS6Rot=[1 0 0;0 1 0;0 0 1]  CS7Pos=[0 0 0]  CS7Rot=[1 0 0;0 1 0;0 0 1]  CS8Pos=[]  CS8Rot=[]  CS9Pos=[]  CS9Rot=[]  CS10Pos=[]  CS10Rot=[]  CS11Pos=[]  CS11Rot=[]  CS12Pos=[]  CS12Rot=[]  CS13Pos=[]  CS13Rot=[]  CS14Pos=[]  CS14Rot=[]  CS15Pos=[]  CS15Rot=[]  CS16Pos=[]  CS16Rot=[]  CS17Pos=[]  CS17Rot=[]  CS18Pos=[]  CS18Rot=[]  CS19Pos=[]  CS19Rot=[]  CS20Pos=[]  CS20Rot=[]
  secondfingerlink-1 : mblibv1/Bodies/Body  DialogController=MECH.DynMechDlgSource  PhysicalDomain=mechanical  SubClassName=Unknown  LeftPortType=workingframe  RightPortType=workingframe  LConnTagsString=CS2  RConnTagsString=CS4|CS3  DialogClass=MechanicalBodyBlock  Mass=0.0053478  MassUnits=kg  InertiaUnits=kg*m^2  Inertia=[6.2632e-008 3.353e-023 1.3973e-023;3.353e-023 4.2402e-007 -4.2564e-025;1.3973e-023 -4.2564e-025 4.4496e-007]  Shape=robot - grip-1 secondfingerlink-1  ShapeDims=[1 1]  ShapeUnits=m  ShapeUse=false  Density=1  DensityUnits=kg/m^3  DensityUse=false  CG=Right$CG$[0.28769 0.13118 0.012778]$WORLD$WORLD$m$[-0.55298 0 0.8332;0 1 0;-0.8332 0 -0.55298]$3x3 Transform$rad$WORLD$false  WorkingFrames=Right$CS4$[0 0 0]$WORLD$WORLD$m$[1 0 0;0 1 0;0 0 1]$3x3 Transform$rad$WORLD$true#Left$CS2$[0.28286 0.13118 0.0054884]$WORLD$WORLD$m$[1 0 0;0 1 0;0 0 1]$3x3 Transform$rad$WORLD$true#Right$CS3$[0.29493 0.13118 0.023689]$WORLD$WORLD$m$[1 0 0;0 1 0;0 0 1]$3x3 Transform$rad$WORLD$true#Right$CS1$[0.29493 0.13118 0.023689]$WORLD$WORLD$m$[1 0 0;0 1 0;0 0 1]$3x3 Transform$rad$WORLD$false  CGPos=[0.28769 0.13118 0.012778]  CGRot=[-0.55298 0 0.8332;0 1 0;-0.8332 0 -0.55298]  CS0Pos=[]  CS0Rot=[]  CS1Pos=[0.29493 0.13118 0.023689]  CS1Rot=[1 0 0;0 1 0;0 0 1]  CS2Pos=[0.28286 0.13118 0.0054884]  CS2Rot=[1 0 0;0 1 0;0 0 1]  CS3Pos=[0.29493 0.13118 0.023689]  CS3Rot=[1 0 0;0 1 0;0 0 1]  CS4Pos=[0 0 0]  CS4Rot=[1 0 0;0 1 0;0 0 1]  CS5Pos=[]  CS5Rot=[]  CS6Pos=[]  CS6Rot=[]  CS7Pos=[]  CS7Rot=[]  CS8Pos=[]  CS8Rot=[]  CS9Pos=[]  CS9Rot=[]  CS10Pos=[]  CS10Rot=[]  CS11Pos=[]  CS11Rot=[]  CS12Pos=[]  CS12Rot=[]  CS13Pos=[]  CS13Rot=[]  CS14Pos=[]  CS14Rot=[]  CS15Pos=[]  CS15Rot=[]  CS16Pos=[]  CS16Rot=[]  CS17Pos=[]  CS17Rot=[]  CS18Pos=[]  CS18Rot=[]  CS19Pos=[]  CS19Rot=[]  CS20Pos=[]  CS20Rot=[]
  secondfingerlink-2 : mblibv1/Bodies/Body  DialogController=MECH.DynMechDlgSource  PhysicalDomain=mechanical  SubClassName=Unknown  LeftPortType=workingframe  RightPortType=workingframe  LConnTagsString=CS2  RConnTagsString=CS4|CS3  DialogClass=MechanicalBodyBlock  Mass=0.0053478  MassUnits=kg  InertiaUnits=kg*m^2  Inertia=[6.2632e-008 3.353e-023 1.3973e-023;3.353e-023 4.2402e-007 -4.2564e-025;1.3973e-023 -4.2564e-025 4.4496e-007]  Shape=robot - grip-1 secondfingerlink-2  ShapeDims=[1 1]  ShapeUnits=m  ShapeUse=false  Density=1  DensityUnits=kg/m^3  DensityUse=false  CG=Right$CG$[0.28769 0.13118 -0.012778]$WORLD$WORLD$m$[-0.55298 0 -0.8332;0 1 0;0.8332 0 -0.55298]$3x3 Transform$rad$WORLD$false  WorkingFrames=Right$CS4$[0 0 0]$WORLD$WORLD$m$[1 0 0;0 1 0;0 0 1]$3x3 Transform$rad$WORLD$true#Left$CS2$[0.28286 0.13118 -0.0054884]$WORLD$WORLD$m$[1 0 0;0 1 0;0 0 1]$3x3 Transform$rad$WORLD$true#Right$CS3$[0.29493 0.13118 -0.023689]$WORLD$WORLD$m$[1 0 0;0 1 0;0 0 1]$3x3 Transform$rad$WORLD$true#Right$CS1$[0.29493 0.13118 -0.023689]$WORLD$WORLD$m$[1 0 0;0 1 0;0 0 1]$3x3 Transform$rad$WORLD$false  CGPos=[0.28769 0.13118 -0.012778]  CGRot=[-0.55298 0 -0.8332;0 1 0;0.8332 0 -0.55298]  CS0Pos=[]  CS0Rot=[]  CS1Pos=[0.29493 0.13118 -0.023689]  CS1Rot=[1 0 0;0 1 0;0 0 1]  CS2Pos=[0.28286 0.13118 -0.0054884]  CS2Rot=[1 0 0;0 1 0;0 0 1]  CS3Pos=[0.29493 0.13118 -0.023689]  CS3Rot=[1 0 0;0 1 0;0 0 1]  CS4Pos=[0 0 0]  CS4Rot=[1 0 0;0 1 0;0 0 1]  CS5Pos=[]  CS5Rot=[]  CS6Pos=[]  CS6Rot=[]  CS7Pos=[]  CS7Rot=[]  CS8Pos=[]  CS8Rot=[]  CS9Pos=[]  CS9Rot=[]  CS10Pos=[]  CS10Rot=[]  CS11Pos=[]  CS11Rot=[]  CS12Pos=[]  CS12Rot=[]  CS13Pos=[]  CS13Rot=[]  CS14Pos=[]  CS14Rot=[]  CS15Pos=[]  CS15Rot=[]  CS16Pos=[]  CS16Rot=[]  CS17Pos=[]  CS17Rot=[]  CS18Pos=[]  CS18Rot=[]  CS19Pos=[]  CS19Rot=[]  CS20Pos=[]  CS20Rot=[]
  Port 1 : PMIOPort  Tag=PMCPort  Port=1  Side=Left
  tag scope: FFL_Left_Pos=global, FFL_Left_Rot=global, FFL_Right_Pos=global, FFL_Right_Rot=global, Meta_Pos=global, Meta_Rot=global, SFL_Left_Pos=global, SFL_Left_Rot=global, SFL_Right_Pos=global, SFL_Right_Rot=global, Tip_Left_Pos=global, Tip_Left_Rot=global, Tip_Right_Pos=global, Tip_Right_Rot=global
  wires:
  Body Sensor/1 -> [FFL_Left_Pos]
  Body Sensor/2 -> [FFL_Left_Rot]
  Body Sensor1/1 -> [Tip_Left_Pos]
  Body Sensor1/2 -> [Tip_Left_Rot]
  Body Sensor2/1 -> [SFL_Left_Pos]
  Body Sensor2/2 -> [SFL_Left_Rot]
  Body Sensor3/1 -> [FFL_Right_Pos]
  Body Sensor3/2 -> [FFL_Right_Rot]
  Body Sensor4/1 -> [SFL_Right_Pos]
  Body Sensor4/2 -> [SFL_Right_Rot]
  Body Sensor5/1 -> [Meta_Pos]
  Body Sensor5/2 -> [Meta_Rot]
  Body Sensor6/1 -> [Tip_Right_Pos]
  Body Sensor6/2 -> [Tip_Right_Rot]
  connections:
  Revolute/LConn1 -- metacarples-1/RConn5
  Revolute/RConn1 -- firstfingerlink-1/LConn1
  Revolute1/LConn1 -- metacarples-1/RConn2
  Revolute1/RConn1 -- firstfingerlinkL-1/LConn1
  Revolute2/LConn1 -- metacarples-1/RConn4
  Revolute2/RConn1 -- secondfingerlink-1/LConn1
  Revolute3/LConn1 -- metacarples-1/RConn3
  Revolute3/RConn1 -- secondfingerlink-2/LConn1
  Revolute4/LConn1 -- firstfingerlink-1/RConn2
  Revolute4/RConn1 -- fingertips-1/LConn2
  Revolute5/LConn1 -- secondfingerlink-1/RConn2
  Revolute5/RConn1 -- fingertips-1/LConn1
  Revolute6/LConn1 -- firstfingerlinkL-1/RConn2
  Revolute6/RConn1 -- fingertips-2/LConn1
  Revolute7/LConn1 -- secondfingerlink-2/RConn2
  Revolute7/RConn1 -- fingertips-2/LConn2
  Port 1/RConn1 -- metacarples-1/LConn1
  metacarples-1/RConn1 -- Body Sensor5/LConn1
  firstfingerlinkL-1/RConn1 -- Body Sensor/LConn1
  secondfingerlink-2/RConn1 -- Body Sensor2/LConn1
  firstfingerlink-1/RConn1 -- Body Sensor3/LConn1
  secondfingerlink-1/RConn1 -- Body Sensor4/LConn1
  fingertips-2/RConn1 -- Body Sensor1/LConn1
  fingertips-1/RConn1 -- Body Sensor6/LConn1
